simulink model "CAM_Example"  (R2021a)
settings: Solver=VariableStepAuto  StartTime=0.0  StopTime=10.0  RelTol=1e-3
libraries: c2xlib x51, simulink x1
settings Model: EnablePacing=on  Creator=User  LastModifiedBy=User

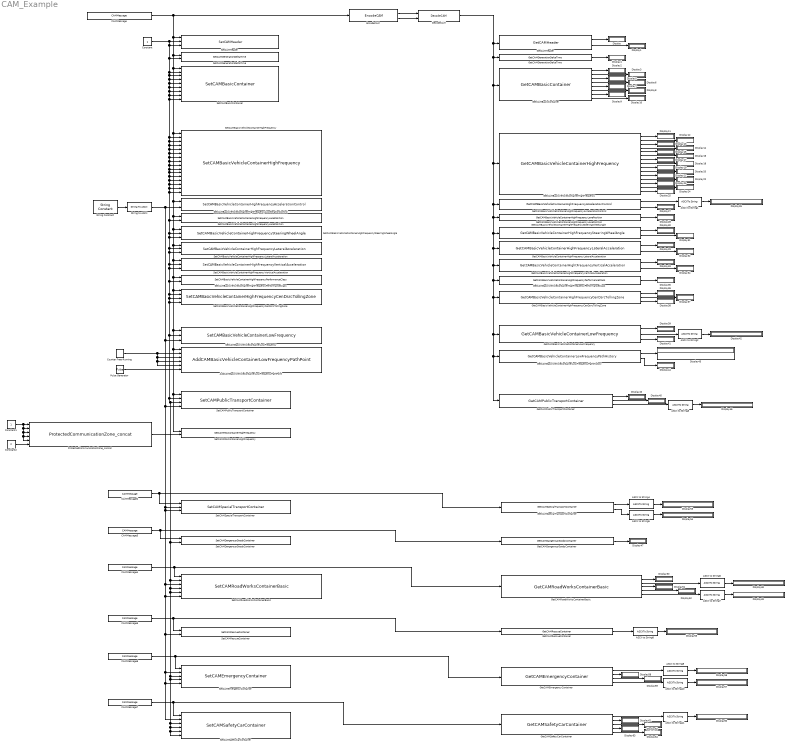
== system CAM_Example ==
  ASCII to String{1..11} (11 alike) : ASCIIToString
  AddCAMBasicVehicleContainerLowFrequencyPathPoint : c2xlib/AddCAMBasicVehicleContainerLowFrequencyPathPoint  SimulateUsing=Code generation
      settings: SourceProductName=C2XLib
  CAMMessage : c2xlib/CAMMessage  StationID=0  HeighFrequencyContainerType=0  SimulateUsing=Code generation
      settings: SourceProductName=C2XLib
  CAMMessage2 : c2xlib/CAMMessage  StationID=3  HeighFrequencyContainerType=0  SimulateUsing=Code generation
      settings: SourceProductName=C2XLib
  CAMMessage3 : c2xlib/CAMMessage  StationID=4  HeighFrequencyContainerType=0  SimulateUsing=Code generation
      settings: SourceProductName=C2XLib
  CAMMessage4 : c2xlib/CAMMessage  StationID=5  HeighFrequencyContainerType=0  SimulateUsing=Code generation
      settings: SourceProductName=C2XLib
  CAMMessage5 : c2xlib/CAMMessage  StationID=6  HeighFrequencyContainerType=0  SimulateUsing=Code generation
      settings: SourceProductName=C2XLib
  CAMMessage6 : c2xlib/CAMMessage  StationID=7  HeighFrequencyContainerType=0  SimulateUsing=Code generation
      settings: SourceProductName=C2XLib
  CAMMessage7 : c2xlib/CAMMessage  StationID=8  HeighFrequencyContainerType=0  SimulateUsing=Code generation
      settings: SourceProductName=C2XLib
  Constant : Constant
  Constant1 : Constant
  Constant2 : Constant  Value=2
  Counter Free-Running : simulink/Sources/Counter Free-Running  NumBits=16  tsamp=1
  DecodeCAM : c2xlib/DecodeCAM  SimulateUsing=Code generation
      settings: SourceProductName=C2XLib
  Display{,1..64} (65 alike) : Display
  EncodeCAM : c2xlib/EncodeCAM  BufferSize=65535  SimulateUsing=Code generation
      settings: SourceProductName=C2XLib
  GetCAMBasicContainer : c2xlib/GetCAMBasicContainer  SimulateUsing=Code generation
      settings: SourceProductName=C2XLib
  GetCAMBasicVehicleContainerHighFrequency : c2xlib/GetCAMBasicVehicleContainerHighFrequency  SimulateUsing=Code generation
      settings: SourceProductName=C2XLib
  GetCAMBasicVehicleContainerHighFrequencyAccelerationControl : c2xlib/GetCAMBasicVehicleContainerHighFrequencyAccelerationControl  BufferSize=32  SimulateUsing=Code generation
      settings: SourceProductName=C2XLib
  GetCAMBasicVehicleContainerHighFrequencyCenDsrcTollingZone : c2xlib/GetCAMBasicVehicleContainerHighFrequencyCenDsrcTollingZone  SimulateUsing=Code generation
      settings: SourceProductName=C2XLib
  GetCAMBasicVehicleContainerHighFrequencyLanePosition : c2xlib/GetCAMBasicVehicleContainerHighFrequencyLanePosition  SimulateUsing=Code generation
      settings: SourceProductName=C2XLib
  GetCAMBasicVehicleContainerHighFrequencyLateralAcceleration : c2xlib/GetCAMBasicVehicleContainerHighFrequencyLateralAcceleration  SimulateUsing=Code generation
      settings: SourceProductName=C2XLib
  GetCAMBasicVehicleContainerHighFrequencyPerformanceClass : c2xlib/GetCAMBasicVehicleContainerHighFrequencyPerformanceClass  SimulateUsing=Code generation
      settings: SourceProductName=C2XLib
  GetCAMBasicVehicleContainerHighFrequencySteeringWheelAngle : c2xlib/GetCAMBasicVehicleContainerHighFrequencySteeringWheelAngle  SimulateUsing=Code generation
      settings: SourceProductName=C2XLib
  GetCAMBasicVehicleContainerHightFrequencyVerticalAcceleration : c2xlib/GetCAMBasicVehicleContainerHightFrequencyVerticalAcceleration  SimulateUsing=Code generation
      settings: SourceProductName=C2XLib
  GetCAMBasicVehicleContainerLowFrequency : c2xlib/GetCAMBasicVehicleContainerLowFrequency  ExteriorLightsSize=32  SimulateUsing=Code generation
      settings: SourceProductName=C2XLib
  GetCAMBasicVehicleContainerLowFrequencyPathHistory : c2xlib/GetCAMBasicVehicleContainerLowFrequencyPathHistory  PathHistorySize=2  SimulateUsing=Code generation
      settings: SourceProductName=C2XLib
  GetCAMDangerousGoodsContainer : c2xlib/GetCAMDangerousGoodsContainer  LightBarSirenInUseSize=1  SpecialTransportTypeSize=1  SimulateUsing=Code generation
      settings: SourceProductName=C2XLib
  GetCAMEmergencyContainer : c2xlib/GetCAMEmergencyContainer  LightBarSirenInUseSize=32  EmergencyPrioritySize=32  SimulateUsing=Code generation
      settings: SourceProductName=C2XLib
  GetCAMGenerationDeltaTime : c2xlib/GetCAMGenerationDeltaTime  SimulateUsing=Code generation
      settings: SourceProductName=C2XLib
  GetCAMHeader : c2xlib/GetCAMHeader  SimulateUsing=Code generation
      settings: SourceProductName=C2XLib
  GetCAMPublicTransportContainer : c2xlib/GetCAMPublicTransportContainer  PtActivationDataSize=32  SimulateUsing=Code generation
      settings: SourceProductName=C2XLib
  GetCAMRescueContainer : c2xlib/GetCAMRescueContainer  LightBarSirenInUseSize=32  SimulateUsing=Code generation
      settings: SourceProductName=C2XLib
  GetCAMRoadWorksContainerBasic : c2xlib/GetCAMRoadWorksContainerBasic  LightBarSirenInUseSize=32  ClosedLaneDrivingLaneStatusSize=32  SimulateUsing=Code generation
      settings: SourceProductName=C2XLib
  GetCAMSafetyCarContainer : c2xlib/GetCAMSafetyCarContainer  LightBarSirenInUseSize=32  SimulateUsing=Code generation
      settings: SourceProductName=C2XLib
  GetCAMSpecialTransportContainer : c2xlib/GetCAMSpecialTransportContainer  LightBarSirenInUseSize=32  SpecialTransportTypeSize=32  SimulateUsing=Code generation
      settings: SourceProductName=C2XLib
  ProtectedCommunicationZone_concat : c2xlib/ProtectedCommunicationZone_concat  SimulateUsing=Code generation
      settings: SourceProductName=C2XLib
  Pulse Generator : DiscretePulseGenerator  PulseType=Time based  PulseWidth=50  PhaseDelay=1
  SetCAMBasicContainer : c2xlib/SetCAMBasicContainer  SimulateUsing=Code generation
      settings: SourceProductName=C2XLib
  SetCAMBasicVehicleContainerHighFrequency : c2xlib/SetCAMBasicVehicleContainerHighFrequency  SimulateUsing=Code generation
      settings: SourceProductName=C2XLib
  SetCAMBasicVehicleContainerHighFrequencyAccelerationControl : c2xlib/SetCAMBasicVehicleContainerHighFrequencyAccelerationControl  SimulateUsing=Code generation
      settings: SourceProductName=C2XLib
  SetCAMBasicVehicleContainerHighFrequencyCenDsrcTollingZone : c2xlib/SetCAMBasicVehicleContainerHighFrequencyCenDsrcTollingZone  SimulateUsing=Code generation
      settings: SourceProductName=C2XLib
  SetCAMBasicVehicleContainerHighFrequencyLanePosition : c2xlib/SetCAMBasicVehicleContainerHighFrequencyLanePosition  SimulateUsing=Code generation
      settings: SourceProductName=C2XLib
  SetCAMBasicVehicleContainerHighFrequencyLateralAcceleration : c2xlib/SetCAMBasicVehicleContainerHighFrequencyLateralAcceleration  SimulateUsing=Code generation
      settings: SourceProductName=C2XLib
  SetCAMBasicVehicleContainerHighFrequencySteeringWheelAngle : c2xlib/SetCAMBasicVehicleContainerHighFrequencySteeringWheelAngle  SimulateUsing=Code generation
      settings: SourceProductName=C2XLib
  SetCAMBasicVehicleContainerHighFrequencyVerticalAcceleration : c2xlib/SetCAMBasicVehicleContainerHighFrequencyVerticalAcceleration  SimulateUsing=Code generation
      settings: SourceProductName=C2XLib
  SetCAMBasicVehicleContainerLowFrequency : c2xlib/SetCAMBasicVehicleContainerLowFrequency  SimulateUsing=Code generation
      settings: SourceProductName=C2XLib
  SetCAMBasicVehivleContainerHighFrequencyPerformanceClass : c2xlib/SetCAMBasicVehivleContainerHighFrequencyPerformanceClass  SimulateUsing=Code generation
      settings: SourceProductName=C2XLib
  SetCAMDangerousGoodsContainer : c2xlib/SetCAMDangerousGoodsContainer  SimulateUsing=Code generation
      settings: SourceProductName=C2XLib
  SetCAMEmergencyContainer : c2xlib/SetCAMEmergencyContainer  SimulateUsing=Code generation
      settings: SourceProductName=C2XLib
  SetCAMGenerationDeltaTime : c2xlib/SetCAMGenerationDeltaTime  SimulateUsing=Code generation
      settings: SourceProductName=C2XLib
  SetCAMHeader : c2xlib/SetCAMHeader  SimulateUsing=Code generation
      settings: SourceProductName=C2XLib
  SetCAMPublicTransportContainer : c2xlib/SetCAMPublicTransportContainer  SimulateUsing=Code generation
      settings: SourceProductName=C2XLib
  SetCAMRSUContainerHighFrequency : c2xlib/SetCAMRSUContainerHighFrequency  ProtectedCommunicationZoneNumber=1  SimulateUsing=Code generation
      settings: SourceProductName=C2XLib
  SetCAMRescueContainer : c2xlib/SetCAMRescueContainer  SimulateUsing=Code generation
      settings: SourceProductName=C2XLib
  SetCAMRoadWorksContainerBasic : c2xlib/SetCAMRoadWorksContainerBasic  SimulateUsing=Code generation
      settings: SourceProductName=C2XLib
  SetCAMSafetyCarContainer : c2xlib/SetCAMSafetyCarContainer  SimulateUsing=Code generation
      settings: SourceProductName=C2XLib
  SetCAMSpecialTransportContainer : c2xlib/SetCAMSpecialTransportContainer  SimulateUsing=Code generation
      settings: SourceProductName=C2XLib
  String Constant : StringConstant  String="\"Byte Array\""
  String to ASCII : StringToASCII
  wires:
  EncodeCAM/2 -> DecodeCAM/2
  EncodeCAM/1 -> DecodeCAM/1
  CAMMessage/1 -> SetCAMRSUContainerHighFrequency/1, SetCAMPublicTransportContainer/1, AddCAMBasicVehicleContainerLowFrequencyPathPoint/1, SetCAMBasicVehicleContainerLowFrequency/1, SetCAMBasicVehicleContainerHighFrequencyCenDsrcTollingZone/1, SetCAMBasicVehivleContainerHighFrequencyPerformanceClass/1, SetCAMBasicVehicleContainerHighFrequencyVerticalAcceleration/1, SetCAMBasicVehicleContainerHighFrequencyLateralAcceleration/1, SetCAMBasicVehicleContainerHighFrequencySteeringWheelAngle/1, SetCAMBasicVehicleContainerHighFrequencyLanePosition/1, SetCAMBasicVehicleContainerHighFrequencyAccelerationControl/1, SetCAMBasicVehicleContainerHighFrequency/1, SetCAMBasicContainer/1, SetCAMGenerationDeltaTime/1, SetCAMHeader/1, EncodeCAM/1
  DecodeCAM/1 -> GetCAMPublicTransportContainer/1, GetCAMBasicVehicleContainerLowFrequencyPathHistory/1, GetCAMBasicVehicleContainerLowFrequency/1, GetCAMBasicVehicleContainerHighFrequencyCenDsrcTollingZone/1, GetCAMBasicVehicleContainerHighFrequencyPerformanceClass/1, GetCAMBasicVehicleContainerHightFrequencyVerticalAcceleration/1, GetCAMBasicVehicleContainerHighFrequencyLateralAcceleration/1, GetCAMBasicVehicleContainerHighFrequencySteeringWheelAngle/1, GetCAMBasicVehicleContainerHighFrequencyLanePosition/1, GetCAMBasicVehicleContainerHighFrequencyAccelerationControl/1, GetCAMBasicVehicleContainerHighFrequency/1, GetCAMBasicContainer/1, GetCAMGenerationDeltaTime/1, GetCAMHeader/1
  GetCAMHeader/2 -> Display1/1
  GetCAMHeader/1 -> Display/1
  GetCAMBasicContainer/2 -> Display3/1
  GetCAMBasicContainer/1 -> Display2/1
  GetCAMGenerationDeltaTime/1 -> Display4/1
  GetCAMBasicContainer/3 -> Display5/1
  GetCAMBasicContainer/4 -> Display6/1
  GetCAMBasicContainer/5 -> Display7/1
  GetCAMBasicContainer/6 -> Display8/1
  GetCAMBasicContainer/7 -> Display9/1
  GetCAMBasicContainer/8 -> Display10/1
  GetCAMBasicVehicleContainerHighFrequency/1 -> Display11/1
  GetCAMBasicVehicleContainerHighFrequency/2 -> Display12/1
  GetCAMBasicVehicleContainerHighFrequency/3 -> Display13/1
  GetCAMBasicVehicleContainerHighFrequency/4 -> Display14/1
  GetCAMBasicVehicleContainerHighFrequency/5 -> Display15/1
  GetCAMBasicVehicleContainerHighFrequency/6 -> Display16/1
  GetCAMBasicVehicleContainerHighFrequency/11 -> Display21/1
  GetCAMBasicVehicleContainerHighFrequency/12 -> Display22/1
  GetCAMBasicVehicleContainerHighFrequency/7 -> Display17/1
  GetCAMBasicVehicleContainerHighFrequency/10 -> Display20/1
  GetCAMBasicVehicleContainerHighFrequency/8 -> Display18/1
  GetCAMBasicVehicleContainerHighFrequency/9 -> Display19/1
  GetCAMBasicVehicleContainerHighFrequency/13 -> Display23/1
  GetCAMBasicVehicleContainerHighFrequency/14 -> Display24/1
  GetCAMBasicVehicleContainerHighFrequency/15 -> Display25/1
  GetCAMBasicVehicleContainerHighFrequencyAccelerationControl/2 -> Display27/1
  GetCAMBasicVehicleContainerHighFrequencyAccelerationControl/1 -> ASCII to String1/1
  GetCAMBasicVehicleContainerHighFrequencyLanePosition/1 -> Display28/1
  GetCAMBasicVehicleContainerHighFrequencySteeringWheelAngle/1 -> Display30/1
  GetCAMBasicVehicleContainerHighFrequencySteeringWheelAngle/2 -> Display31/1
  GetCAMBasicVehicleContainerHighFrequencyLateralAcceleration/2 -> Display32/1
  GetCAMBasicVehicleContainerHighFrequencyLateralAcceleration/1 -> Display29/1
  GetCAMBasicVehicleContainerHightFrequencyVerticalAcceleration/2 -> Display34/1
  GetCAMBasicVehicleContainerHightFrequencyVerticalAcceleration/1 -> Display33/1
  GetCAMBasicVehicleContainerHighFrequencyPerformanceClass/1 -> Display35/1
  GetCAMBasicVehicleContainerHighFrequencyCenDsrcTollingZone/1 -> Display36/1
  GetCAMBasicVehicleContainerHighFrequencyCenDsrcTollingZone/2 -> Display37/1
  GetCAMBasicVehicleContainerHighFrequencyCenDsrcTollingZone/3 -> Display38/1
  GetCAMBasicVehicleContainerLowFrequency/1 -> Display39/1
  GetCAMBasicVehicleContainerLowFrequency/2 -> ASCII to String2/1
  GetCAMBasicVehicleContainerLowFrequency/3 -> Display41/1
  GetCAMBasicVehicleContainerLowFrequencyPathHistory/1 -> Display43/1
  GetCAMBasicVehicleContainerLowFrequencyPathHistory/2 -> Display44/1
  Pulse Generator/1 -> AddCAMBasicVehicleContainerLowFrequencyPathPoint/6
  String Constant/1 -> String to ASCII/1
  ASCII to String1/1 -> Display26/1
  ASCII to String2/1 -> Display42/1
  Counter Free-Running/1 -> AddCAMBasicVehicleContainerLowFrequencyPathPoint/2, AddCAMBasicVehicleContainerLowFrequencyPathPoint/3, AddCAMBasicVehicleContainerLowFrequencyPathPoint/4, AddCAMBasicVehicleContainerLowFrequencyPathPoint/5
  GetCAMPublicTransportContainer/1 -> Display40/1
  GetCAMPublicTransportContainer/2 -> Display45/1
  GetCAMPublicTransportContainer/3 -> ASCII to String3/1
  ASCII to String3/1 -> Display46/1
  CAMMessage2/1 -> SetCAMSpecialTransportContainer/1, GetCAMSpecialTransportContainer/1
  GetCAMSpecialTransportContainer/1 -> ASCII to String4/1
  ASCII to String4/1 -> Display53/1
  GetCAMSpecialTransportContainer/2 -> ASCII to String5/1
  ASCII to String5/1 -> Display54/1
  CAMMessage3/1 -> GetCAMDangerousGoodsContainer/1, SetCAMDangerousGoodsContainer/1
  Constant/1 -> SetCAMSafetyCarContainer/6, SetCAMSafetyCarContainer/5, SetCAMSafetyCarContainer/4, SetCAMSafetyCarContainer/3, SetCAMEmergencyContainer/4, SetCAMEmergencyContainer/3, SetCAMRoadWorksContainerBasic/5, SetCAMRoadWorksContainerBasic/4, SetCAMRoadWorksContainerBasic/2, SetCAMDangerousGoodsContainer/2, SetCAMPublicTransportContainer/3, SetCAMPublicTransportContainer/2, SetCAMBasicVehicleContainerLowFrequency/2, SetCAMBasicVehicleContainerHighFrequencyCenDsrcTollingZone/4, SetCAMBasicVehicleContainerHighFrequencyCenDsrcTollingZone/3, SetCAMBasicVehicleContainerHighFrequencyCenDsrcTollingZone/2, SetCAMBasicVehivleContainerHighFrequencyPerformanceClass/2, SetCAMBasicVehicleContainerHighFrequencyVerticalAcceleration/3, SetCAMBasicVehicleContainerHighFrequencyVerticalAcceleration/2, SetCAMBasicVehicleContainerHighFrequencyLateralAcceleration/3, SetCAMBasicVehicleContainerHighFrequencyLateralAcceleration/2, SetCAMBasicVehicleContainerHighFrequencySteeringWheelAngle/3, SetCAMBasicVehicleContainerHighFrequencySteeringWheelAngle/2, SetCAMBasicVehicleContainerHighFrequencyLanePosition/2, SetCAMBasicVehicleContainerHighFrequency/16, SetCAMBasicVehicleContainerHighFrequency/15, SetCAMBasicVehicleContainerHighFrequency/14, SetCAMBasicVehicleContainerHighFrequency/13, SetCAMBasicVehicleContainerHighFrequency/12, SetCAMBasicVehicleContainerHighFrequency/11, SetCAMBasicVehicleContainerHighFrequency/10, SetCAMBasicVehicleContainerHighFrequency/9, SetCAMBasicVehicleContainerHighFrequency/8, SetCAMBasicVehicleContainerHighFrequency/7, SetCAMBasicVehicleContainerHighFrequency/6, SetCAMBasicVehicleContainerHighFrequency/5, SetCAMBasicVehicleContainerHighFrequency/4, SetCAMBasicVehicleContainerHighFrequency/3, SetCAMBasicVehicleContainerHighFrequency/2, SetCAMBasicContainer/9, SetCAMBasicContainer/8, SetCAMBasicContainer/7, SetCAMBasicContainer/6, SetCAMBasicContainer/5, SetCAMBasicContainer/4, SetCAMBasicContainer/3, SetCAMBasicContainer/2, SetCAMGenerationDeltaTime/2, SetCAMHeader/3, SetCAMHeader/2
  GetCAMDangerousGoodsContainer/1 -> Display47/1
  CAMMessage4/1 -> GetCAMRoadWorksContainerBasic/1, SetCAMRoadWorksContainerBasic/1
  ASCII to String6/1 -> Display48/1
  ASCII to String7/1 -> Display49/1
  GetCAMRoadWorksContainerBasic/5 -> ASCII to String7/1
  GetCAMRoadWorksContainerBasic/2 -> ASCII to String6/1
  GetCAMRoadWorksContainerBasic/1 -> Display50/1
  GetCAMRoadWorksContainerBasic/4 -> Display52/1
  GetCAMRoadWorksContainerBasic/3 -> Display51/1
  CAMMessage5/1 -> GetCAMRescueContainer/1, SetCAMRescueContainer/1
  ASCII to String8/1 -> Display55/1
  GetCAMRescueContainer/1 -> ASCII to String8/1
  CAMMessage6/1 -> GetCAMEmergencyContainer/1, SetCAMEmergencyContainer/1
  String to ASCII/1 -> SetCAMSafetyCarContainer/2, SetCAMEmergencyContainer/5, SetCAMEmergencyContainer/2, SetCAMRescueContainer/2, SetCAMRoadWorksContainerBasic/6, SetCAMRoadWorksContainerBasic/3, SetCAMSpecialTransportContainer/3, SetCAMSpecialTransportContainer/2, SetCAMPublicTransportContainer/4, SetCAMBasicVehicleContainerLowFrequency/3, SetCAMBasicVehicleContainerHighFrequencyAccelerationControl/2
  ASCII to String9/1 -> Display56/1
  ASCII to String10/1 -> Display57/1
  GetCAMEmergencyContainer/4 -> ASCII to String10/1
  GetCAMEmergencyContainer/1 -> ASCII to String9/1
  GetCAMEmergencyContainer/2 -> Display58/1
  GetCAMEmergencyContainer/3 -> Display59/1
  CAMMessage7/1 -> GetCAMSafetyCarContainer/1, SetCAMSafetyCarContainer/1
  ASCII to String11/1 -> Display60/1
  GetCAMSafetyCarContainer/1 -> ASCII to String11/1
  GetCAMSafetyCarContainer/2 -> Display61/1
  GetCAMSafetyCarContainer/3 -> Display62/1
  GetCAMSafetyCarContainer/4 -> Display63/1
  GetCAMSafetyCarContainer/5 -> Display64/1
  ProtectedCommunicationZone_concat/1 -> SetCAMRSUContainerHighFrequency/2
  Constant1/1 -> ProtectedCommunicationZone_concat/5, ProtectedCommunicationZone_concat/4, ProtectedCommunicationZone_concat/3, ProtectedCommunicationZone_concat/2, ProtectedCommunicationZone_concat/1
  Constant2/1 -> ProtectedCommunicationZone_concat/6
